simulink model "Message_eg2_2018a"  (R2018a)
settings: Solver=VariableStepAuto  StartTime=0.0  StopTime=10.0  RelTol=1e-3
settings Model: Creator=86188  LastModifiedBy=86188

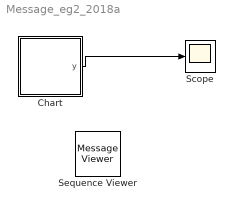
== system Message_eg2_2018a ==
  Chart : Stateflow chart  TreatAsAtomicUnit=on
  Scope : Scope
  Sequence Viewer : MessageViewer
  wires:
  Chart/1(y) -> Scope/1

== stateflow chart Message_eg2_2018a/Chart ==
  state A
    en:
    f("en_A");
    M1.data=4;
    M.data=3;
    M2.data=3;
    send(M1);
    send(M);
    send(M1);
  state B
    en:
    f("en_B");
    y=1;
  state C
    en:f("en_C");
    y=2;
  state D
    en:f("en_D");
  (default) -> A
  A -> B : M[M1.data==4]
  B -> C : M1
  C -> D : M1
  data: s function_input; M local; y output; M1 local; M2 local
  function f(s):
    | function f(s)
    |   fprintf(s+"\n");
